simulink model "synchronous_buck"  (R2022b)
settings: Solver=VariableStepAuto  StartTime=0.0  StopTime=10  RelTol=1e-3
model workspace (MAT data in the model file):
  D = 0.3
libraries: spsDiodeLib x14, spsACVoltageSourceLib x6, spsSeriesRLCBranchLib x5, spsVoltageMeasurementLib x4, spsCurrentMeasurementLib x3, spsDCVoltageSourceLib x3, spsMosfetLib x3, spsControlledVoltageSourceLib x2, spsDCMachineLib x2, simulink x2, sps_lib x1
settings Model: Creator=alman  LastModifiedBy=alman
settings SolverCC: ZeroCrossAlgorithm=Adaptive
settings DebuggingCC: IgnoredZcDiagnostic=none

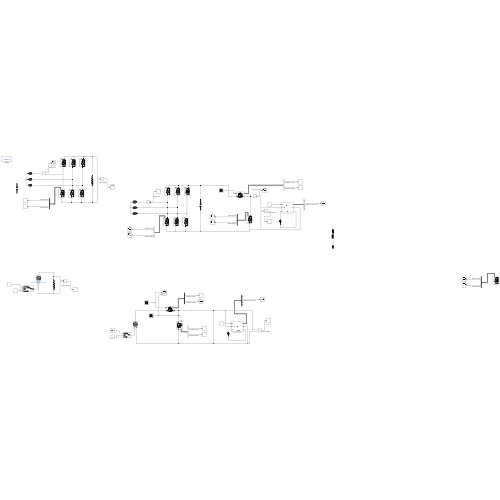
[thumbnail: Simulink's stored preview of the top-level diagram]
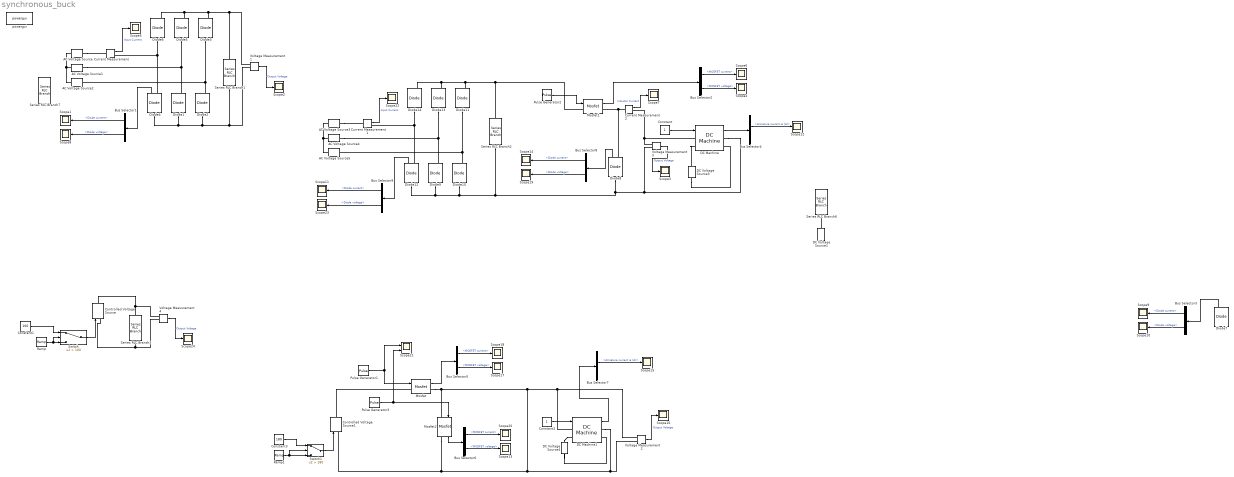
== system synchronous_buck ==
  AC Voltage Source : spsACVoltageSourceLib/AC Voltage Source  Amplitude=100*sqrt(2)  Phase=0  Frequency=50  SampleTime=0  Measurements=None  BusType=swing  Pref=10e3  Qref=0  Qmin=-inf  Qmax=+inf
  AC Voltage Source1 : spsACVoltageSourceLib/AC Voltage Source  Amplitude=100*sqrt(2)  Phase=-120  Frequency=50  SampleTime=0  Measurements=None  BusType=swing  Pref=10e3  Qref=0  Qmin=-inf  Qmax=+inf
  AC Voltage Source2 : spsACVoltageSourceLib/AC Voltage Source  Amplitude=100*sqrt(2)  Phase=-240  Frequency=50  SampleTime=0  Measurements=None  BusType=swing  Pref=10e3  Qref=0  Qmin=-inf  Qmax=+inf
  AC Voltage Source3 : spsACVoltageSourceLib/AC Voltage Source  Amplitude=100*sqrt(2)  Phase=0  Frequency=50  SampleTime=0  Measurements=None  BusType=swing  Pref=10e3  Qref=0  Qmin=-inf  Qmax=+inf
  AC Voltage Source4 : spsACVoltageSourceLib/AC Voltage Source  Amplitude=100*sqrt(2)  Phase=-120  Frequency=50  SampleTime=0  Measurements=None  BusType=swing  Pref=10e3  Qref=0  Qmin=-inf  Qmax=+inf
  AC Voltage Source5 : spsACVoltageSourceLib/AC Voltage Source  Amplitude=100*sqrt(2)  Phase=-240  Frequency=50  SampleTime=0  Measurements=None  BusType=swing  Pref=10e3  Qref=0  Qmin=-inf  Qmax=+inf
  Bus Selector{1,3,8..9} (4 alike) : BusSelector  OutputSignals=Diode current,Diode voltage
  Bus Selector2 : BusSelector  OutputSignals=MOSFET current,MOSFET voltage
  Bus Selector4 : BusSelector  OutputSignals=Speed wm (rad/s),Armature current ia (A),Field current if (A),Electrical torque Te (n m)
  Bus Selector5 : BusSelector  OutputSignals=MOSFET current,MOSFET voltage
  Bus Selector6 : BusSelector  OutputSignals=MOSFET current,MOSFET voltage
  Bus Selector7 : BusSelector  OutputSignals=Speed wm (rad/s),Armature current ia (A),Field current if (A),Electrical torque Te (n m)
  Constant : Constant
  Constant1 : Constant  Value=100
  Constant2 : Constant
  Constant3 : Constant  Value=180
  Controlled Voltage Source : spsControlledVoltageSourceLib/Controlled Voltage Source  Initialize=on  Source_Type=AC  Amplitude=0  Phase=0  Frequency=50  Measurements=None
  Controlled Voltage Source1 : spsControlledVoltageSourceLib/Controlled Voltage Source  Initialize=on  Source_Type=DC  Amplitude=0  Phase=0  Frequency=0  Measurements=None
  Current Measurement : spsCurrentMeasurementLib/Current Measurement  PhasorSimulation=off  OutputType=Complex  PSBequivalent=0
  Current Measurement1 : spsCurrentMeasurementLib/Current Measurement  PhasorSimulation=off  OutputType=Complex  PSBequivalent=0
  Current Measurement2 : spsCurrentMeasurementLib/Current Measurement  PhasorSimulation=off  OutputType=Complex  PSBequivalent=0
  DC Machine : spsDCMachineLib/DC Machine  PresetModel=No  MechanicalLoad=Torque TL  FieldType=Wound  ShowDetailedParameters=on  MeasurementBus=off  RLa="[ 1.07  24.5e-3]"  RLf="[ 240  120]"  Laf=1.8  MachineConstant=Torque constant (N.m/A)  Ke=1.8  Kt=1.8  J=1  Bm=0  Tf=0  w0=0  Ifinit=0.74999999925978  TsPowergui=0  TsBlock=-1
  DC Machine1 : spsDCMachineLib/DC Machine  PresetModel=No  MechanicalLoad=Torque TL  FieldType=Wound  ShowDetailedParameters=on  MeasurementBus=off  RLa="[ 1.07  24.5e-3]"  RLf="[ 240  120]"  Laf=1.8  MachineConstant=Torque constant (N.m/A)  Ke=1.8  Kt=1.8  J=1  Bm=0  Tf=0  w0=0  Ifinit=0.75  TsPowergui=0  TsBlock=-1
  DC Voltage Source1 : spsDCVoltageSourceLib/DC Voltage Source  Amplitude=120  Measurements=None
  DC Voltage Source3 : spsDCVoltageSourceLib/DC Voltage Source  Amplitude=180  Measurements=None
  DC Voltage Source4 : spsDCVoltageSourceLib/DC Voltage Source  Amplitude=180  Measurements=None
  Diode{1..14} (14 alike) : spsDiodeLib/Diode  Ron=0.001  Lon=0  Vf=0.8  IC=0  UseSnubber=0  Rs=500  Cs=250e-9  Measurements=on
  Mosfet : spsMosfetLib/Mosfet  Ron=0.1  Lon=0  Rd=0.01  Vfd=0  IC=0  Rs=1e5  Cs=inf  Measurements=on
  Mosfet1 : spsMosfetLib/Mosfet  Ron=0.1  Lon=0  Rd=0.01  Vfd=0  IC=0  Rs=1e5  Cs=inf  Measurements=on
  Mosfet2 : spsMosfetLib/Mosfet  Ron=0.1  Lon=0  Rd=0.01  Vfd=0  IC=0  Rs=1e5  Cs=inf  Measurements=on
  Pulse Generator1 : DiscretePulseGenerator  PulseType=Time based  Amplitude=1000  Period=1/7800  PulseWidth=D*100
  Pulse Generator2 : DiscretePulseGenerator  PulseType=Time based  Amplitude=5  Period=1/7800  PulseWidth=50
  Pulse Generator3 : DiscretePulseGenerator  PulseType=Time based  Amplitude=1000  Period=1/7800  PulseWidth=(1-D)*100  PhaseDelay=(1/7800)*(D)
  Ramp : simulink/Sources/Ramp  slope=10  start=0  InitialOutput=0
  Ramp1 : simulink/Sources/Ramp  slope=10  start=0  InitialOutput=0
  Scope{1..20,22..24} (23 alike) : Scope
  Scope21 : Scope  NumInputPorts=2
  Series RLC Branch1 : spsSeriesRLCBranchLib/Series RLC Branch  LConnTagsString=__new0  RConnTagsString=__new0  BranchType=R  Resistance=50  Inductance=1e-3  SetiL0=off  InitialCurrent=0  Capacitance=100e-6  Setx0=off  InitialVoltage=0  Measurements=None
  Series RLC Branch2 : spsSeriesRLCBranchLib/Series RLC Branch  LConnTagsString=__new0  RConnTagsString=__new0  BranchType=C  Resistance=1  Inductance=1e-3  SetiL0=off  InitialCurrent=0  Capacitance=990e-6  Setx0=off  InitialVoltage=0  Measurements=None
  Series RLC Branch3 : spsSeriesRLCBranchLib/Series RLC Branch  LConnTagsString=__new0  RConnTagsString=__new0  BranchType=R  Resistance=100  Inductance=1e-3  SetiL0=off  InitialCurrent=0  Capacitance=100e-6  Setx0=off  InitialVoltage=0  Measurements=None
  Series RLC Branch6 : spsSeriesRLCBranchLib/Series RLC Branch  LConnTagsString=__new0  RConnTagsString=__new0  BranchType=RL  Resistance=1.07  Inductance=24.5e-3  SetiL0=off  InitialCurrent=0  Capacitance=1e-6  Setx0=off  InitialVoltage=0  Measurements=None
  Series RLC Branch7 : spsSeriesRLCBranchLib/Series RLC Branch  LConnTagsString=__new0  RConnTagsString=__new0  BranchType=C  Resistance=1  Inductance=1e-3  SetiL0=off  InitialCurrent=0  Capacitance=100e-6  Setx0=off  InitialVoltage=0  Measurements=None
  Switch : Switch  Criteria=u2 > Threshold  Threshold=100  SaturateOnIntegerOverflow=off  InputSameDT=off
  Switch1 : Switch  Criteria=u2 > Threshold  Threshold=180  SaturateOnIntegerOverflow=off  InputSameDT=off
  Voltage Measurement{1..4} (4 alike) : spsVoltageMeasurementLib/Voltage Measurement  PhasorSimulation=off  OutputType=Complex  PSBequivalent=0
  powergui : sps_lib/powergui  Priority=1  SimulationMode=Continuous  SampleTime=50e-6  frequency=60  Iterations=50  frequencyindice=0  Pbase=100e6  ErrMax=1e-4  UnitsV=kV  UnitsW=MW  buscounter=0  FunctionMessages=off  echomessages=off  EnableUseOfTLC=off  CurrentSourceSwitches=off  DisableSnubberDevices=off  DisableRonSwitches=off  DisableVfSwitches=off  DisplayEquations=off  AutomaticDiscreteSolvers=off  SolverType=Tustin/Backward Euler (TBE)  Interpol=off  ExternalGateDelay=off  methode=off  Ts=100  x0status=blocks  SPID=on  SwTol=0  HookPort=off  NonlinearTolerance=1e-4  nMaxIteration=100  ContinueOnMaxIteration=off  RestoreLinks=warning  ResistiveCurrentMeasurement=off  Frange=[0:2:500]  Ylog=off  Xlog=on  ShowGrid=off  save=off  variable=ZData  structure=0  ZoomFFT=off  StartTime=0.0  cycles=1  DisplayStyle=1  fundamental=60  FreqAxis=off  MaxFrequency=1000  frequencyindicesteady=1  RmsSteady=1  display=off
  wires:
  Voltage Measurement1/1 -> Scope2/1  "Output Voltage"
  Pulse Generator2/1 -> Mosfet1/1
  Voltage Measurement3/1 -> Scope3/1  "Output Voltage"
  Current Measurement/1 -> Scope5/1  "Input Current"
  Bus Selector1/1 -> Scope1/1  "<Diode current>"
  Bus Selector1/2 -> Scope8/1  "<Diode voltage>"
  Diode4/1 -> Bus Selector1/1
  Mosfet1/1 -> Bus Selector2/1
  Bus Selector2/1 -> Scope6/1  "<MOSFET current>"
  Bus Selector2/2 -> Scope4/1  "<MOSFET voltage>"
  Current Measurement2/1 -> Scope7/1  "Inductor Current"
  Constant/1 -> DC Machine/1
  DC Machine/1 -> Bus Selector4/1
  Bus Selector4/2 -> Scope12/1  "<Armature current ia (A)>"
  Constant3/1 -> Switch1/1
  Switch1/1 -> Controlled Voltage Source1/1
  Ramp1/1 -> Switch1/3, Switch1/2
  Bus Selector7/2 -> Scope15/1  "<Armature current ia (A)>"
  DC Machine1/1 -> Bus Selector7/1
  Constant2/1 -> DC Machine1/1
  Bus Selector5/2 -> Scope17/1  "<MOSFET voltage>"
  Bus Selector5/1 -> Scope18/1  "<MOSFET current>"
  Mosfet/1 -> Bus Selector5/1
  Voltage Measurement2/1 -> Scope16/1  "Output Voltage"
  Pulse Generator1/1 -> Mosfet/1, Scope21/1
  Pulse Generator3/1 -> Mosfet2/1, Scope21/2
  Mosfet2/1 -> Bus Selector6/1
  Bus Selector6/1 -> Scope20/1  "<MOSFET current>"
  Bus Selector6/2 -> Scope13/1  "<MOSFET voltage>"
  Bus Selector3/2 -> Scope10/1  "<Diode voltage>"
  Bus Selector3/1 -> Scope9/1  "<Diode current>"
  Diode7/1 -> Bus Selector3/1
  Diode8/1 -> Bus Selector8/1
  Bus Selector8/2 -> Scope19/1  "<Diode voltage>"
  Bus Selector8/1 -> Scope14/1  "<Diode current>"
  Switch/1 -> Controlled Voltage Source/1
  Ramp/1 -> Switch/2, Switch/3
  Constant1/1 -> Switch/1
  Diode12/1 -> Bus Selector9/1
  Bus Selector9/2 -> Scope23/1  "<Diode voltage>"
  Bus Selector9/1 -> Scope11/1  "<Diode current>"
  Current Measurement1/1 -> Scope22/1  "Input Current"
  Voltage Measurement4/1 -> Scope24/1  "Output Voltage"
  connections:
  AC Voltage Source1/RConn1 -- Diode5/LConn1 -- Diode1/RConn1
  Diode6/LConn1 -- Current Measurement/RConn1 -- Diode4/RConn1
  AC Voltage Source/LConn1 -- AC Voltage Source1/LConn1 -- AC Voltage Source2/LConn1
  AC Voltage Source/RConn1 -- Current Measurement/LConn1
  AC Voltage Source2/RConn1 -- Diode3/LConn1 -- Diode2/RConn1
  Voltage Measurement1/LConn2 -- Series RLC Branch1/RConn1 -- Diode2/LConn1 -- Diode4/LConn1 -- Diode1/LConn1
  Voltage Measurement1/LConn1 -- Series RLC Branch1/LConn1 -- Diode5/RConn1 -- Diode6/RConn1 -- Diode3/RConn1
  Current Measurement2/LConn1 -- Mosfet1/RConn1 -- Diode8/RConn1
  Voltage Measurement3/LConn1 -- Current Measurement2/RConn1 -- DC Machine/LConn1
  DC Machine/LConn2 -- DC Voltage Source3/RConn1
  DC Voltage Source3/LConn1 -- DC Machine/RConn2
  DC Voltage Source1/RConn1 -- Series RLC Branch6/RConn1
  DC Machine1/LConn1 -- Voltage Measurement2/LConn1 -- DC Machine1/RConn1 -- Voltage Measurement2/LConn2 -- Mosfet2/RConn1 -- Controlled Voltage Source1/LConn1 -- Mosfet/RConn1 -- Mosfet2/LConn1
  DC Machine1/LConn2 -- DC Voltage Source4/RConn1
  Mosfet/LConn1 -- Controlled Voltage Source1/RConn1
  DC Voltage Source4/LConn1 -- DC Machine1/RConn2
  AC Voltage Source4/RConn1 -- Diode9/RConn1 -- Diode13/LConn1
  Current Measurement1/RConn1 -- Diode12/RConn1 -- Diode14/LConn1
  AC Voltage Source3/LConn1 -- AC Voltage Source5/LConn1 -- AC Voltage Source4/LConn1
  AC Voltage Source5/RConn1 -- Diode10/RConn1 -- Diode11/LConn1
  Series RLC Branch2/RConn1 -- Diode9/LConn1 -- Diode12/LConn1 -- Diode10/LConn1 -- Diode8/LConn1 -- Voltage Measurement3/LConn2 -- DC Machine/RConn1
  Diode13/RConn1 -- Diode14/RConn1 -- Mosfet1/LConn1 -- Series RLC Branch2/LConn1 -- Diode11/RConn1
  AC Voltage Source3/RConn1 -- Current Measurement1/LConn1
  Controlled Voltage Source/RConn1 -- Voltage Measurement4/LConn1 -- Series RLC Branch3/LConn1
  Controlled Voltage Source/LConn1 -- Voltage Measurement4/LConn2 -- Series RLC Branch3/RConn1
